simulink model "bille_synthese"  (R2019a)
settings: Solver=ode45  StartTime=0.0  StopTime=20  RelTol=1e-3  EnableMultiTasking=on
values from neighbouring files (symbols this model uses):
  f = 7E-5    (= 7e-05)    [BallOnBeam.m]
  J = 4.6E-5    (= 4.6e-05)    [BallOnBeam.m]
  k = 0.026    [BallOnBeam.m]
  k1 = 7    [BallOnBeam.m]
  k2 = 28.65    [BallOnBeam.m]
  k3 = 0.0159    [BallOnBeam.m]
  kb = 6.1    [BallOnBeam.m]
  ki = 1.6    [BallOnBeam.m]
  kp = nm*J*wndes^2/(k2*k*ki)    (= 27.0462934428)    [BallOnBeam.m]
  kpi = rm*tii*ki/taudesi    (= 1.6)    [BallOnBeam.m]
  kv = (2*xides*J*wndes - f)/(kp*ki*k*k3)    (= 0.093347474441)    [BallOnBeam.m]
  lm = 0.001    [BallOnBeam.m]
  nm = 960    [BallOnBeam.m]
  r0 = x(3)    [BallOnBeam.m]
  r1 = x(4)    [BallOnBeam.m]
  r2 = x(5)    [BallOnBeam.m]
  rm = 0.33    [BallOnBeam.m]
  s1 = x(2)    [BallOnBeam.m]
  Te = 0.2    [BallOnBeam.m]
  tii = 0.5*lm/rm    (= 0.00151515151515)    [BallOnBeam.m]
settings Model: ExtModeTrigMode=oneshot  ExtModeArmWhenConnect=off  Creator=khennouh  LastModifiedBy=DELL
settings DataIOCC: SaveFormat=Array  SignalLoggingSaveFormat=ModelDataLogs  ReturnWorkspaceOutputs=off
settings OptimizationCC: BlockReduction=off  BooleanDataType=off
settings DebuggingCC: SaveWithParameterizedLinksMsg=none  UnderspecifiedInitializationDetection=Classic  MergeDetectMultiDrivingBlocksExec=none  SignalResolutionControl=TryResolveAllWithWarning  MultiTaskDSMMsg=warning  MultiTaskCondExecSysMsg=none  PregeneratedLibrarySubsystemCodeDiagnostic=none  ArithmeticOperatorsInVariantConditions=warning
settings HardwareCC: TargetUnknown=on
settings ModelReferenceCC: PropagateSignalLabelsOutOfModel=off
settings SFSimCC: SimUseLocalCustomCode=off
settings RTWCC: RTWUseLocalCustomCode=off
settings CodeAppCC: StateflowObjectComments=on
settings GRTTargetCC: TargetLangStandard=C89/C90 (ANSI)  CombineOutputUpdateFcns=off  GRTInterface=on

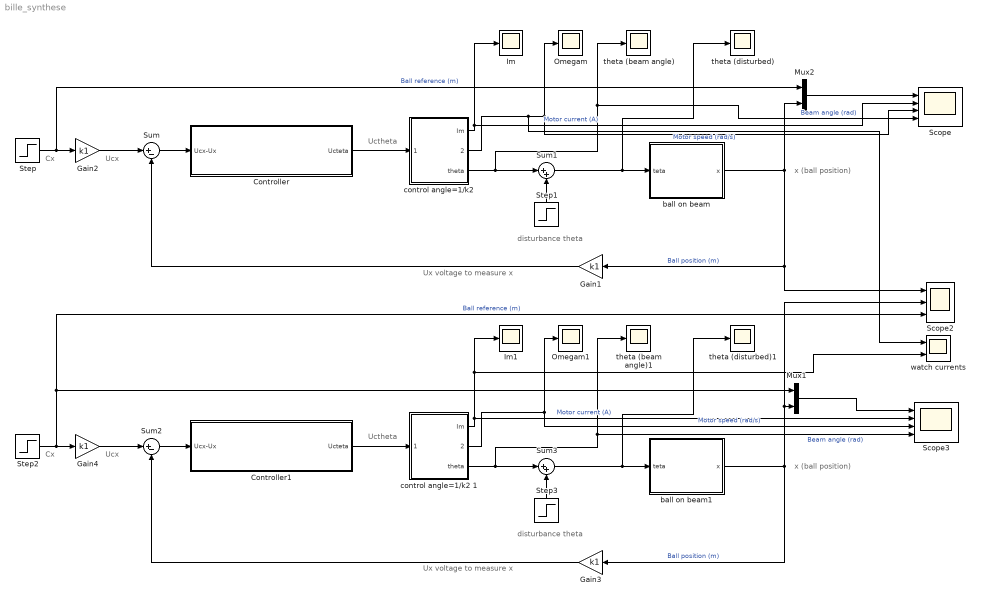
== system bille_synthese ==
  note: disturbance theta
  note: Uctheta
  note: x (ball position)
  note: Ucx
  note: Ux voltage to measure x
  note: Cx
  note: Cx
  note: disturbance theta
  note: Ux voltage to measure x
  note: x (ball position)
  note: Uctheta
  note: Ucx
  Controller : Subsystem
  Controller1 : Subsystem
  Gain{1..4} (4 alike) : Gain  Gain=k1  SaturateOnIntegerOverflow=on  OutDataTypeStr=Inherit: Same as input  ParamDataTypeStr=Inherit: Same as input
  Im : Scope
  Im1 : Scope
  Mux1 : Mux  Inputs=2
  Mux2 : Mux  Inputs=2
  Omegam : Scope
  Omegam1 : Scope
  Scope : Scope  NumInputPorts=4
  Scope2 : Scope  NumInputPorts=3
  Scope3 : Scope  NumInputPorts=4
  Step : Step  After=0.1  SampleTime=0
  Step1 : Step  Time=10  After=1*pi/180  SampleTime=0
  Step2 : Step  After=0.1  SampleTime=0
  Step3 : Step  Time=10  After=1*pi/180  SampleTime=0
  Sum : Sum  Inputs=|+-  SaturateOnIntegerOverflow=on  InputSameDT=on  OutDataTypeStr=Inherit: Same as first input
  Sum1 : Sum  Inputs=|++  SaturateOnIntegerOverflow=on  InputSameDT=on  OutDataTypeStr=Inherit: Same as first input
  Sum2 : Sum  Inputs=|+-  SaturateOnIntegerOverflow=on  InputSameDT=on  OutDataTypeStr=Inherit: Same as first input
  Sum3 : Sum  Inputs=|++  SaturateOnIntegerOverflow=on  InputSameDT=on  OutDataTypeStr=Inherit: Same as first input
  ball on beam : Subsystem
  ball on beam1 : Subsystem
  "control angle=1/k2 " : Subsystem
  control angle=1/k2 1 : Subsystem
  theta (beam angle) : Scope
  theta (beam angle)1 : Scope
  theta (disturbed) : Scope
  theta (disturbed)1 : Scope
  "watch currents " : Scope  NumInputPorts=2
  wires:
  "control angle=1/k2 "/1(Im) -> Im/1, Scope/2  "Motor current (A)"
  "control angle=1/k2 "/2(omega) -> "watch currents "/1, Omegam/1, Scope/3  "Motor speed (rad/s)"
  Gain1/1 -> Sum/2
  Gain2/1 -> Sum/1
  Step/1 -> Mux2/1, Gain2/1  "Ball reference (m)"
  Step1/1 -> Sum1/2
  Mux2/1 -> Scope/1
  "control angle=1/k2 "/3(theta) -> Scope/4, theta (beam angle)/1, Sum1/1  "Beam angle (rad)"
  ball on beam/1(x) -> Mux2/2, Scope2/1, Gain1/1  "Ball position (m)"
  Sum1/1 -> theta (disturbed)/1, ball on beam/1(teta)
  Sum/1 -> Controller/1(Ucx-Ux)
  Controller/1(Ucteta) -> "control angle=1/k2 "/1(Uctheta)
  control angle=1/k2 1/1(Im) -> "watch currents "/2, Im1/1, Scope3/2  "Motor current (A)"
  Gain3/1 -> Sum2/2
  control angle=1/k2 1/3(theta) -> theta (beam angle)1/1, Scope3/4, Sum3/1  "Beam angle (rad)"
  Controller1/1(Ucteta) -> control angle=1/k2 1/1(Uctheta)
  Sum2/1 -> Controller1/1(Ucx-Ux)
  Sum3/1 -> theta (disturbed)1/1, ball on beam1/1(teta)
  Mux1/1 -> Scope3/1
  Step2/1 -> Scope2/3, Mux1/1, Gain4/1  "Ball reference (m)"
  Step3/1 -> Sum3/2
  control angle=1/k2 1/2(omega) -> Omegam1/1, Scope3/3  "Motor speed (rad/s)"
  Gain4/1 -> Sum2/1
  ball on beam1/1(x) -> Scope2/2, Mux1/2, Gain3/1  "Ball position (m)"

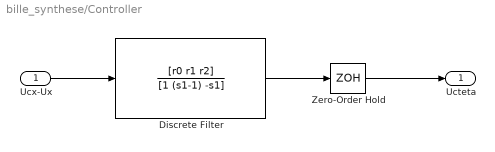
== system bille_synthese/Controller ==
  Ucx-Ux : Inport
  Discrete Filter : DiscreteFilter  Numerator=[r0 r1 r2]  Denominator=[1 (s1-1) -s1]  SampleTime=Te
  Zero-Order Hold : ZeroOrderHold  SampleTime=-1
  Ucteta : Outport
  wires:
  Ucx-Ux/1 -> Discrete Filter/1
  Zero-Order Hold/1 -> Ucteta/1
  Discrete Filter/1 -> Zero-Order Hold/1

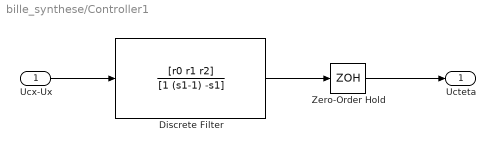
== system bille_synthese/Controller1 ==
  Ucx-Ux : Inport
  Discrete Filter : DiscreteFilter  Numerator=[r0 r1 r2]  Denominator=[1 (s1-1) -s1]  SampleTime=Te
  Zero-Order Hold : ZeroOrderHold  SampleTime=-1
  Ucteta : Outport
  wires:
  Ucx-Ux/1 -> Discrete Filter/1
  Zero-Order Hold/1 -> Ucteta/1
  Discrete Filter/1 -> Zero-Order Hold/1

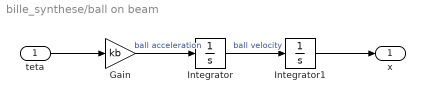
== system bille_synthese/ball on beam ==
  teta : Inport
  Gain : Gain  Gain=kb
  Integrator : Integrator
  Integrator1 : Integrator
  x : Outport
  wires:
  Integrator/1 -> Integrator1/1  "ball velocity"
  Integrator1/1 -> x/1
  teta/1 -> Gain/1
  Gain/1 -> Integrator/1  "ball acceleration"

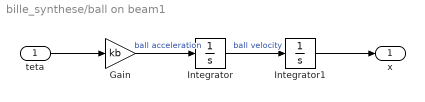
== system bille_synthese/ball on beam1 ==
  teta : Inport
  Gain : Gain  Gain=kb
  Integrator : Integrator
  Integrator1 : Integrator
  x : Outport
  wires:
  Integrator/1 -> Integrator1/1  "ball velocity"
  Integrator1/1 -> x/1
  teta/1 -> Gain/1
  Gain/1 -> Integrator/1  "ball acceleration"

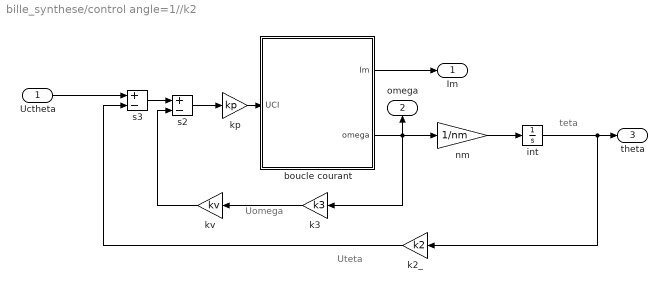
== system bille_synthese/control angle=1//k2  ==
  note: Uomega
  note: teta
  note: Uteta
  Uctheta : Inport
  boucle courant : Subsystem
  int : Integrator
  k2_ : Gain  Gain=k2  SaturateOnIntegerOverflow=on  OutDataTypeStr=Inherit: Same as input  ParamDataTypeStr=Inherit: Same as input
  k3 : Gain  Gain=k3  SaturateOnIntegerOverflow=on  OutDataTypeStr=Inherit: Same as input  ParamDataTypeStr=Inherit: Same as input
  kp : Gain  Gain=kp  SaturateOnIntegerOverflow=on  OutDataTypeStr=Inherit: Same as input  ParamDataTypeStr=Inherit: Same as input
  kv : Gain  Gain=kv  SaturateOnIntegerOverflow=on  OutDataTypeStr=Inherit: Same as input  ParamDataTypeStr=Inherit: Same as input
  nm : Gain  Gain=1/nm  SaturateOnIntegerOverflow=on  OutDataTypeStr=Inherit: Same as input  ParamDataTypeStr=Inherit: Same as input
  s2 : Sum  Inputs=+-  SaturateOnIntegerOverflow=on  InputSameDT=on  OutDataTypeStr=Inherit: Same as first input
  s3 : Sum  Inputs=+-  SaturateOnIntegerOverflow=on  InputSameDT=on  OutDataTypeStr=Inherit: Same as first input
  Im : Outport
  omega : Outport  Port=2
  theta : Outport  Port=3
  wires:
  kp/1 -> boucle courant/1(UCI)
  s2/1 -> kp/1
  s3/1 -> s2/1
  nm/1 -> int/1
  boucle courant/2(omega) -> nm/1, k3/1, omega/1
  k3/1 -> kv/1
  kv/1 -> s2/2
  int/1 -> k2_/1, theta/1
  k2_/1 -> s3/2
  boucle courant/1(Im) -> Im/1
  Uctheta/1 -> s3/1

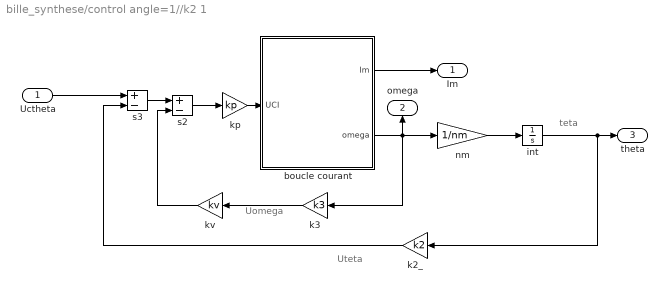
== system bille_synthese/control angle=1//k2 1 ==
  note: Uomega
  note: teta
  note: Uteta
  Uctheta : Inport
  boucle courant : Subsystem
  int : Integrator
  k2_ : Gain  Gain=k2  SaturateOnIntegerOverflow=on  OutDataTypeStr=Inherit: Same as input  ParamDataTypeStr=Inherit: Same as input
  k3 : Gain  Gain=k3  SaturateOnIntegerOverflow=on  OutDataTypeStr=Inherit: Same as input  ParamDataTypeStr=Inherit: Same as input
  kp : Gain  Gain=kp  SaturateOnIntegerOverflow=on  OutDataTypeStr=Inherit: Same as input  ParamDataTypeStr=Inherit: Same as input
  kv : Gain  Gain=kv  SaturateOnIntegerOverflow=on  OutDataTypeStr=Inherit: Same as input  ParamDataTypeStr=Inherit: Same as input
  nm : Gain  Gain=1/nm  SaturateOnIntegerOverflow=on  OutDataTypeStr=Inherit: Same as input  ParamDataTypeStr=Inherit: Same as input
  s2 : Sum  Inputs=+-  SaturateOnIntegerOverflow=on  InputSameDT=on  OutDataTypeStr=Inherit: Same as first input
  s3 : Sum  Inputs=+-  SaturateOnIntegerOverflow=on  InputSameDT=on  OutDataTypeStr=Inherit: Same as first input
  Im : Outport
  omega : Outport  Port=2
  theta : Outport  Port=3
  wires:
  kp/1 -> boucle courant/1(UCI)
  s2/1 -> kp/1
  s3/1 -> s2/1
  nm/1 -> int/1
  boucle courant/2(omega) -> nm/1, k3/1, omega/1
  k3/1 -> kv/1
  kv/1 -> s2/2
  int/1 -> k2_/1, theta/1
  k2_/1 -> s3/2
  boucle courant/1(Im) -> Im/1
  Uctheta/1 -> s3/1

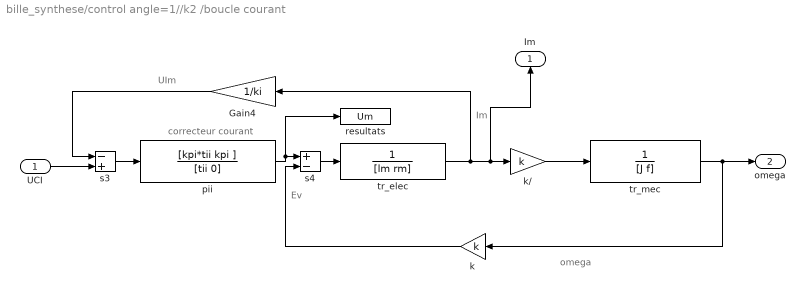
== system bille_synthese/control angle=1//k2 /boucle courant ==
  note: correcteur courant
  note: Im
  note: Ev
  note: UIm
  note: omega
  UCI : Inport
  Gain4 : Gain  Gain=1/ki  SaturateOnIntegerOverflow=on  OutDataTypeStr=Inherit: Same as input  ParamDataTypeStr=Inherit: Same as input
  k : Gain  Gain=k  SaturateOnIntegerOverflow=on  OutDataTypeStr=Inherit: Same as input  ParamDataTypeStr=Inherit: Same as input
  "k/ " : Gain  Gain=k  SaturateOnIntegerOverflow=on  OutDataTypeStr=Inherit: Same as input  ParamDataTypeStr=Inherit: Same as input
  pii : TransferFcn  Numerator=[kpi*tii kpi ]  Denominator=[tii 0]
  resultats : ToWorkspace  VariableName=Um
      settings: MaxDataPoints=20000
  s3 : Sum  Inputs=-+  SaturateOnIntegerOverflow=on  InputSameDT=on  OutDataTypeStr=Inherit: Same as first input
  s4 : Sum  Inputs=+-  SaturateOnIntegerOverflow=on  InputSameDT=on  OutDataTypeStr=Inherit: Same as first input
  tr_elec : TransferFcn  Denominator=[lm rm]
  tr_mec : TransferFcn  Denominator=[J f]
  Im : Outport
  omega : Outport  Port=2
  wires:
  s4/1 -> tr_elec/1
  Gain4/1 -> s3/1
  s3/1 -> pii/1
  k/1 -> s4/2
  "k/ "/1 -> tr_mec/1
  tr_mec/1 -> k/1, omega/1
  UCI/1 -> s3/2
  pii/1 -> s4/1, resultats/1
  tr_elec/1 -> Gain4/1, "k/ "/1, Im/1

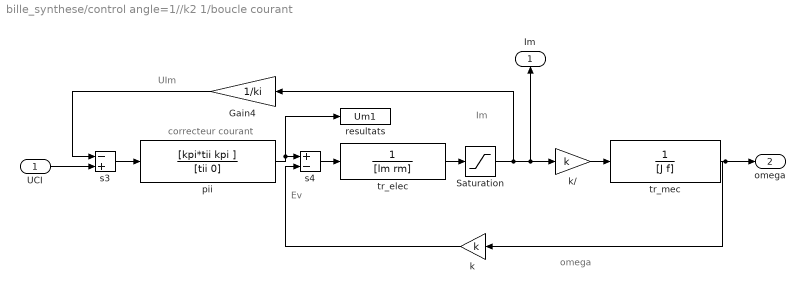
== system bille_synthese/control angle=1//k2 1/boucle courant ==
  note: correcteur courant
  note: Im
  note: Ev
  note: UIm
  note: omega
  UCI : Inport
  Gain4 : Gain  Gain=1/ki  SaturateOnIntegerOverflow=on  OutDataTypeStr=Inherit: Same as input  ParamDataTypeStr=Inherit: Same as input
  Saturation : Saturate  UpperLimit=400  LowerLimit=-400  LinearizeAsGain=off
  k : Gain  Gain=k  SaturateOnIntegerOverflow=on  OutDataTypeStr=Inherit: Same as input  ParamDataTypeStr=Inherit: Same as input
  "k/ " : Gain  Gain=k  SaturateOnIntegerOverflow=on  OutDataTypeStr=Inherit: Same as input  ParamDataTypeStr=Inherit: Same as input
  pii : TransferFcn  Numerator=[kpi*tii kpi ]  Denominator=[tii 0]
  resultats : ToWorkspace  VariableName=Um1
      settings: MaxDataPoints=20000
  s3 : Sum  Inputs=-+  SaturateOnIntegerOverflow=on  InputSameDT=on  OutDataTypeStr=Inherit: Same as first input
  s4 : Sum  Inputs=+-  SaturateOnIntegerOverflow=on  InputSameDT=on  OutDataTypeStr=Inherit: Same as first input
  tr_elec : TransferFcn  Denominator=[lm rm]
  tr_mec : TransferFcn  Denominator=[J f]
  Im : Outport
  omega : Outport  Port=2
  wires:
  s4/1 -> tr_elec/1
  Gain4/1 -> s3/1
  s3/1 -> pii/1
  k/1 -> s4/2
  "k/ "/1 -> tr_mec/1
  tr_mec/1 -> k/1, omega/1
  UCI/1 -> s3/2
  pii/1 -> s4/1, resultats/1
  tr_elec/1 -> Saturation/1
  Saturation/1 -> Gain4/1, Im/1, "k/ "/1
